simulink subsystem "DifferentialDriveDynamic"  (R2024b)
settings: Solver=VariableStepAuto  StartTime=0.0  StopTime=10.0  RelTol=1e-3
model mask{L=32, J=32, M=13, R=120, max_speed=[-Inf Inf], max_accel=[-Inf Inf]}
  mask prompts: L "Distance Between Wheels (m)"; J "Inertia (kg*m^2)"; M "Mass (kg)"; R "Radio of wheel (m)"; max_speed "Max speed (m/s)"; max_accel "Max acceleration(m/s^2)"
settings Model: Creator=marti  LastModifiedBy=marti

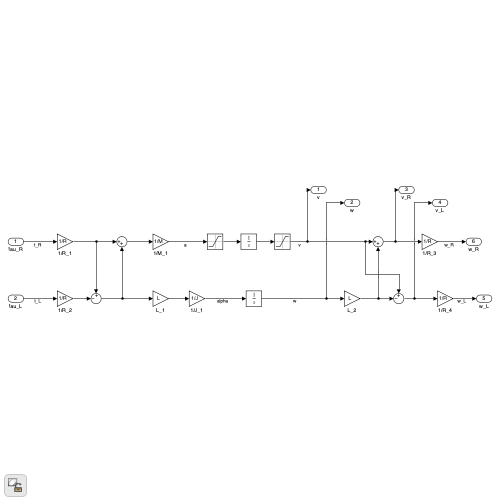
[thumbnail: Simulink's stored preview of the top-level diagram]
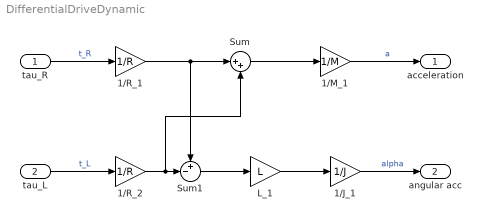
== system DifferentialDriveDynamic ==
  tau_R : Inport
  tau_L : Inport  Port=2
  1/J_1 : Gain  Gain=1/J
  1/M_1 : Gain  Gain=1/M
  1/R_1 : Gain  Gain=1/R
  1/R_2 : Gain  Gain=1/R
  L_1 : Gain  Gain=L
  Sum : Sum  Inputs=|++
  Sum1 : Sum  Inputs=+-|
  acceleration : Outport
  angular acc : Outport  Port=2
  wires:
  tau_R/1 -> 1/R_1/1  "t_R"
  tau_L/1 -> 1/R_2/1  "t_L"
  1/R_1/1 -> Sum1/1, Sum/1
  1/R_2/1 -> Sum1/2, Sum/2
  Sum/1 -> 1/M_1/1
  Sum1/1 -> L_1/1
  L_1/1 -> 1/J_1/1
  1/M_1/1 -> acceleration/1  "a"
  1/J_1/1 -> angular acc/1  "alpha"
